simulink model "task2"  (R2024a)
settings: Solver=VariableStepAuto  StartTime=0.0  StopTime=10.0  RelTol=1e-3
undefined symbols (not defined in the file): B_g_bar, F_bar, ss_gen, ss_gen_disc, T
settings Model: Creator=vladislav  LastModifiedBy=lalayants

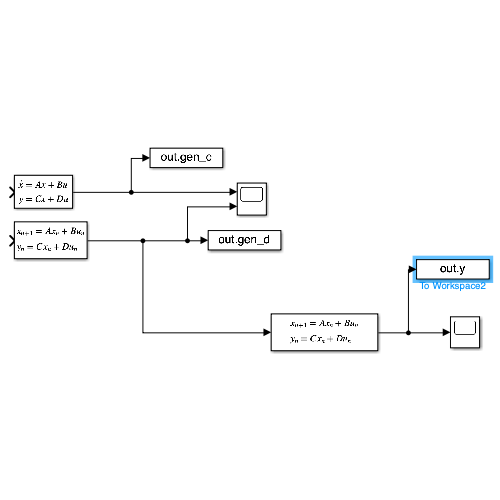
[thumbnail: Simulink's stored preview of the top-level diagram]
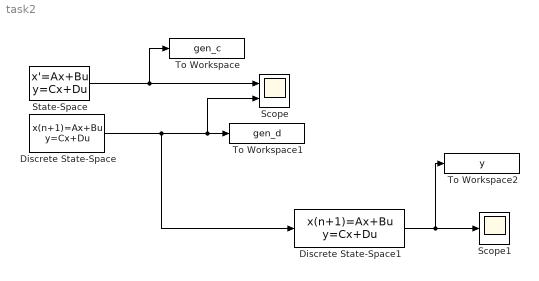
== system task2 ==
  Discrete State-Space : DiscreteStateSpace  A=ss_gen_disc.A  B=ss_gen_disc.B  C=ss_gen_disc.C  D=ss_gen_disc.D  InitialCondition=[0 1]  SampleTime=T
  Discrete State-Space1 : DiscreteStateSpace  A=F_bar  B=B_g_bar  C=[0 0 1 0]  D=0  InitialCondition=[1 1 1 1]  SampleTime=T
  Scope : Scope  NumInputPorts=2
  Scope1 : Scope
  State-Space : StateSpace  A=ss_gen.A  B=ss_gen.B  C=ss_gen.C  D=ss_gen.D  InitialCondition=[0 1]
  To Workspace : ToWorkspace  VariableName=gen_c  SaveFormat=Timeseries  SampleTime=-1
  To Workspace1 : ToWorkspace  VariableName=gen_d  SaveFormat=Timeseries  SampleTime=-1
  To Workspace2 : ToWorkspace  VariableName=y  SaveFormat=Timeseries  SampleTime=-1
  wires:
  State-Space/1 -> Scope/1, To Workspace/1
  Discrete State-Space/1 -> Discrete State-Space1/1, To Workspace1/1, Scope/2
  Discrete State-Space1/1 -> To Workspace2/1, Scope1/1
